simulink subsystem "Motor2022"  (R2022b)
settings: Solver=VariableStepAuto  StartTime=0.0  StopTime=10.0  RelTol=1e-3
model mask{kw=62.8, km=16e-3, motor_nominal_voltage=24, vis_friction_coef_motor=0.1, L=0.00035, R=10, J_motor=5e-07}
settings Model: Creator=mrrom  LastModifiedBy=romav
settings OptimizationCC: ReuseModelBlockBuffer=on

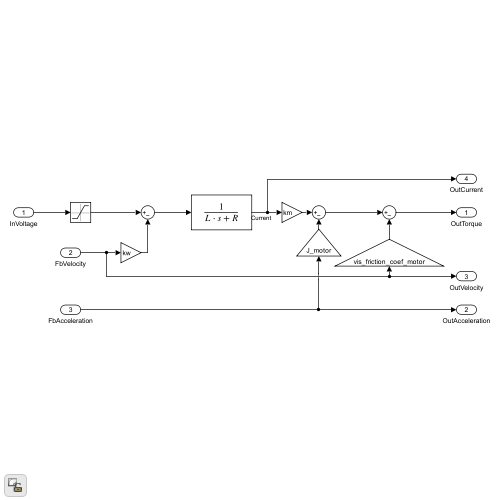
[thumbnail: Simulink's stored preview of the top-level diagram]
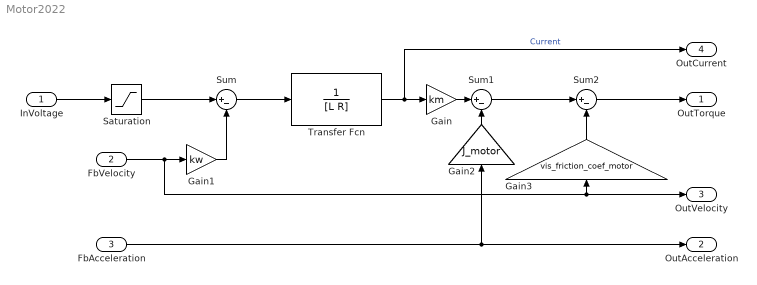
== system Motor2022 ==
  InVoltage : Inport
  FbVelocity : Inport  Port=2
  FbAcceleration : Inport  Port=3
  Gain : Gain  Gain=km
  Gain1 : Gain  Gain=kw
  Gain2 : Gain  Gain=J_motor
  Gain3 : Gain  Gain=vis_friction_coef_motor
  Saturation : Saturate  UpperLimit=motor_nominal_voltage  LowerLimit=-motor_nominal_voltage
  Sum : Sum  Inputs=|+-
  Sum1 : Sum  Inputs=|+-
  Sum2 : Sum  Inputs=|+-
  Transfer Fcn : TransferFcn  Denominator=[L R]
  OutTorque : Outport
  OutAcceleration : Outport  Port=2
  OutVelocity : Outport  Port=3
  OutCurrent : Outport  Port=4
  wires:
  Gain3/1 -> Sum2/2
  Transfer Fcn/1 -> Gain/1, OutCurrent/1  "Current"
  InVoltage/1 -> Saturation/1
  Sum/1 -> Transfer Fcn/1
  Sum2/1 -> OutTorque/1
  FbVelocity/1 -> Gain1/1, Gain3/1, OutVelocity/1
  FbAcceleration/1 -> Gain2/1, OutAcceleration/1
  Gain/1 -> Sum1/1
  Sum1/1 -> Sum2/1
  Gain2/1 -> Sum1/2
  Gain1/1 -> Sum/2
  Saturation/1 -> Sum/1
